simulink model "FullFMS_2026_02_17_V0_3_8"  (R2025b)
settings: Solver=ode23tb  StartTime=0.0  StopTime=inf  MaxStep=0.1  RelTol=1e-2
PreLoadFcn:
  | load("BUS_CONFIG.mat")
libraries: opcualib x8
(part 4 of 4)

== matlab function FullFMS_2026_02_17_V0_3_8/Control_20 ==
  data: u1 input; u2 input; u3 input; u4 input; u5 input; u6 input; u7 input; u8 input; u9 input; u10 input; u11 input; u12 input; C_24_CRoute_In output; C_25_CRoute_In output; C_26_CRoute_In output; C_27_CRoute_In output; C_28_CRoute_In output; C_29_CRoute_In output; C_24_Request output; C_24_CartDel output; C_24_CRoute_Out output; C_25_Request output; C_25_CartDel output; C_25_CRoute_Out output; C_26_Request output; C_26_CartDel output; C_26_CRoute_Out output; C_27_Request output; C_27_CartDel output; C_27_CRoute_Out output; C_28_Request output; C_28_CartDel output; C_28_CRoute_Out output; C_29_Request output; C_29_CartDel output; C_29_CRoute_Out output; u13 input; u14 input; u15 input; u16 input; u17 input; u18 input; u19 input; u20 input; u21 input; u22 input; u23 input; u24 input
function [C_24_CRoute_In,C_25_CRoute_In,C_26_CRoute_In,C_27_CRoute_In,...
C_28_CRoute_In,C_29_CRoute_In,C_24_Request,C_24_CartDel,C_24_CRoute_Out,...
C_25_Request,C_25_CartDel,C_25_CRoute_Out,C_26_Request,C_26_CartDel,...
C_26_CRoute_Out,C_27_Request,C_27_CartDel,C_27_CRoute_Out,C_28_Request,...
C_28_CartDel,C_28_CRoute_Out,C_29_Request,C_29_CartDel,C_29_CRoute_Out]...
= fcn_Control(u1,u2,u3,u4,u5,u6,u7,u8,u9,u10,u11,u12,u13,u14,u15,u16,...
u17,u18,u19,u20,u21,u22,u23,u24)

C_24_CRoute_In = u1;
C_25_CRoute_In = u2;
C_26_CRoute_In = u3;
C_27_CRoute_In = u4;
C_28_CRoute_In = u5;
C_29_CRoute_In = u6;
C_24_Request = u7;
C_24_CartDel = u8;
C_24_CRoute_Out = u9;
C_25_Request = u10;
C_25_CartDel = u11;
C_25_CRoute_Out = u12;
C_26_Request = u13;
C_26_CartDel = u14;
C_26_CRoute_Out = u15;
C_27_Request = u16;
C_27_CartDel = u17;
C_27_CRoute_Out = u18;
C_28_Request = u19;
C_28_CartDel = u20;
C_28_CRoute_Out = u21;
C_29_Request = u22;
C_29_CartDel = u23;
C_29_CRoute_Out = u24;

== matlab function FullFMS_2026_02_17_V0_3_8/Feedback_20 ==
  data: u1 input; F_22_Led_On output; u2 input; u3 input; u4 input; u5 input; u6 input; u7 input; u8 input; u9 input; F_22_Led_Off output; F_22_Conveyor output; F_24_Release_FB output; F_25_Release_FB output; F_26_Release_FB output; F_27_Release_FB output; F_28_Release_FB output; F_29_Release_FB output
function [F_22_Led_On,F_22_Led_Off,F_22_Conveyor,F_24_Release_FB,...
    F_25_Release_FB,F_26_Release_FB,F_27_Release_FB,F_28_Release_FB,...
    F_29_Release_FB] = fcn_Feedback(u1,u2,u3,u4,u5,u6,u7,u8,u9)

F_22_Led_On = u1;
F_22_Led_Off = u2;
F_22_Conveyor = u3;
F_24_Release_FB = u4;
F_25_Release_FB = u5;
F_26_Release_FB = u6;
F_27_Release_FB = u7;
F_28_Release_FB = u8;
F_29_Release_FB = u9;

== matlab function FullFMS_2026_02_17_V0_3_8/Sensors_20 ==
  data: u1 input; O_20_On output; u2 input; u3 input; u4 input; u5 input; u6 input; u7 input; u8 input; u9 input; u10 input; u11 input; u12 input; u13 input; u14 input; u15 input; u16 input; u17 input; u18 input; u19 input; u20 input; u21 input; u22 input; u23 input; u24 input; u25 input; u26 input; u27 input; u28 input; u29 input; u30 input; u31 input; u32 input; u33 input; O_20_Off output; O_20_Controler_On output; O_24_Cart_Stat output; O_24_Cart_Next output; O_24_Optic output; O_24_Count output; O_24_Pist_Bck output; O_25_Cart_Stat output; O_25_Cart_Next output; O_25_Optic output; O_25_Count output; O_25_Pist_Back output; O_26_Cart_Stat output; O_26_Cart_Next output; O_26_Optic output; O_26_Count output; O_26_Pist_Back output; O_27_Cart_Stat output; O_27_Cart_Next output; O_27_Optic output; O_27_Count output; O_27_Pist_Back output; O_28_Cart_Stat output; O_28_Cart_Next output; O_28_Optic output; O_28_Count output; O_28_Pist_Back output; O_29_Cart_Stat output; O_29_Cart_Next output; O_29_Optic output; O_29_Count output; O_29_Pist_Back output
function [O_20_On,O_20_Off,O_20_Controler_On,...
    O_24_Cart_Stat,O_24_Cart_Next,O_24_Optic,O_24_Count,O_24_Pist_Bck,...
    O_25_Cart_Stat,O_25_Cart_Next,O_25_Optic,O_25_Count,O_25_Pist_Back,...
    O_26_Cart_Stat,O_26_Cart_Next,O_26_Optic,O_26_Count,O_26_Pist_Back,...
    O_27_Cart_Stat,O_27_Cart_Next,O_27_Optic,O_27_Count,O_27_Pist_Back,...
    O_28_Cart_Stat,O_28_Cart_Next,O_28_Optic,O_28_Count,O_28_Pist_Back,...
    O_29_Cart_Stat,O_29_Cart_Next,O_29_Optic,O_29_Count,O_29_Pist_Back...
    ] = fcn_Sensors(u1,u2,u3,u4,u5,u6,u7,u8,u9,u10,u11,u12,u13,u14,...
    u15,u16,u17,u18,u19,u20,u21,u22,u23,u24,u25,u26,u27,u28,u29,u30,...
    u31,u32,u33)

O_20_On            = u1;
O_20_Off           = u2;
O_20_Controler_On  = u3;

O_24_Cart_Stat     = u4;
O_24_Cart_Next     = u5;
O_24_Optic         = u6;
O_24_Count         = u7;
O_24_Pist_Bck      = u8;

O_25_Cart_Stat     = u9;
O_25_Cart_Next     = u10;
O_25_Optic         = u11;
O_25_Count         = u12;
O_25_Pist_Back     = u13;

O_26_Cart_Stat     = u14;
O_26_Cart_Next     = u15;
O_26_Optic         = u16;
O_26_Count         = u17;
O_26_Pist_Back     = u18;

O_27_Cart_Stat     = u19;
O_27_Cart_Next     = u20;
O_27_Optic         = u21;
O_27_Count         = u22;
O_27_Pist_Back     = u23;

O_28_Cart_Stat     = u24;
O_28_Cart_Next     = u25;
O_28_Optic         = u26;
O_28_Count         = u27;
O_28_Pist_Back     = u28;

O_29_Cart_Stat     = u29;
O_29_Cart_Next     = u30;
O_29_Optic         = u31;
O_29_Count         = u32;
O_29_Pist_Back     = u33;

== matlab function FullFMS_2026_02_17_V0_3_8/AS-i_50 ==
  data: u1 input; u2 input; u3 input; u4 input; u5 input; u6 input; u7 input; u8 input; u9 input; u10 input; u11 input; u12 input; A_54_Request output; A_54_No_Cart output; A_54_Cart_Full output; A_54_CRoute_Out output; A_53_SortCartID output; A_54_Cart_Stat output; A_54_Cart_Next output; A_54_Optic output; A_54_Count output; A_54_Pist_Bck output; A_54_Release_FB output; A_54_CRoute_In output
function [A_54_Request, A_54_No_Cart, A_54_Cart_Full, A_54_CRoute_Out,...
A_53_SortCartID, A_54_Cart_Stat, A_54_Cart_Next, A_54_Optic, A_54_Count,...
A_54_Pist_Bck, A_54_Release_FB, A_54_CRoute_In]...
= fcn_Asi(u1,u2,u3,u4,u5,u6,u7,u8,u9,u10,u11,u12)

A_54_Request = u1;
A_54_No_Cart = u2;
A_54_Cart_Full = u3;
A_54_CRoute_Out = u4;
A_53_SortCartID = u5;
A_54_Cart_Stat = u6;
A_54_Cart_Next = u7;
A_54_Optic = u8;
A_54_Count = u9;
A_54_Pist_Bck = u10;
A_54_Release_FB = u11;
A_54_CRoute_In = u12;

== matlab function FullFMS_2026_02_17_V0_3_8/Control_50 ==
  data: u1 input; C_55_Initialization output; u2 input; u3 input; u4 input; u5 input; C_55_PD_Sort output; C_52_Profibus output; C_55_Start output; C_55_Cart2Del output
function [C_55_Initialization,C_55_PD_Sort,C_52_Profibus,...
    C_55_Start,C_55_Cart2Del] = fcn_Control(u1,u2,u3,u4,u5)

C_55_Initialization = u1;
C_55_PD_Sort = u2;
C_52_Profibus = u3;
C_55_Start = u4;
C_55_Cart2Del = u5;

== matlab function FullFMS_2026_02_17_V0_3_8/Feedback_50 ==
  data: u1 input; F_52_Claw_2_Del output; u2 input; u3 input; u4 input; u5 input; u6 input; u7 input; u8 input; u9 input; u10 input; u11 input; u12 input; F_52_Claw_2_Cart output; F_52_Claw_Down output; F_52_Close_Claw output; F_53_Led_Start output; F_53_Led_Reset output; F_53_Led_Extra1 output; F_53_Led_Extra2 output; F_53_Panel_O4 output; F_53_Panel_O5 output; F_53_Panel_O6 output; F_53_Panel_O7 output
function [F_52_Claw_2_Del,F_52_Claw_2_Cart,F_52_Claw_Down,...
    F_52_Close_Claw,F_53_Led_Start,F_53_Led_Reset,F_53_Led_Extra1,...
    F_53_Led_Extra2,F_53_Panel_O4,F_53_Panel_O5,F_53_Panel_O6,...
    F_53_Panel_O7] = fcn_Feedback(u1,u2,u3,u4,u5,u6,u7,u8,u9,u10,u11,u12)

F_52_Claw_2_Del = u1;
F_52_Claw_2_Cart = u2;
F_52_Claw_Down = u3;
F_52_Close_Claw = u4;
F_53_Led_Start = u5;
F_53_Led_Reset = u6;
F_53_Led_Extra1 = u7;
F_53_Led_Extra2 = u8;
F_53_Panel_O4 = u9;
F_53_Panel_O5 = u10;
F_53_Panel_O6 = u11;
F_53_Panel_O7 = u12;

== matlab function FullFMS_2026_02_17_V0_3_8/Sensors_50 ==
  data: u1 input; O_50_Part_Reserve output; u2 input; u3 input; u4 input; u5 input; u6 input; u7 input; u8 input; u9 input; u10 input; u11 input; u12 input; u13 input; u14 input; u15 input; O_50_Claw_Cart output; O_50_Claw_Del output; O_50_Claw_Reserve output; O_50_Claw_Low output; O_50_Claw_High output; O_50_Part_in_Claw output; O_51_Start output; O_51_Stop output; O_51_Key_Pos output; O_51_Reset output; O_51_Panel_I4 output; O_51_Panel_I5 output; O_51_Panel_I6 output; O_51_Panel_I7 output
function [O_50_Part_Reserve,O_50_Claw_Cart,O_50_Claw_Del,...
    O_50_Claw_Reserve,O_50_Claw_Low,O_50_Claw_High,O_50_Part_in_Claw,...
    O_51_Start,O_51_Stop,O_51_Key_Pos,O_51_Reset,O_51_Panel_I4,...
    O_51_Panel_I5,O_51_Panel_I6,O_51_Panel_I7] = fcn_Sensors(u1,u2,u3,u4,...
    u5,u6,u7,u8,u9,u10,u11,u12,u13,u14,u15)

O_50_Part_Reserve = u1;
O_50_Claw_Cart = u2;
O_50_Claw_Del = u3;
O_50_Claw_Reserve = u4;
O_50_Claw_Low = u5;
O_50_Claw_High = u6;
O_50_Part_in_Claw = u7;
O_51_Start = u8;
O_51_Stop = u9;
O_51_Key_Pos = u10;
O_51_Reset = u11;
O_51_Panel_I4 = u12;
O_51_Panel_I5 = u13;
O_51_Panel_I6 = u14;
O_51_Panel_I7 = u15;

== matlab function FullFMS_2026_02_17_V0_3_8/AS-i_90 ==
  data: u1 input; A_94_Request output; u2 input; u3 input; u4 input; u5 input; u6 input; u7 input; u8 input; u9 input; A_94_No_Cart output; A_94_Cart_Full output; A_94_CRoute_Out output; A_93_ProcCartID output; A_94_Cart_Stat output; A_94_Cart_Next output; A_94_Optic output; A_94_Count output; A_94_Pist_Bck output; A_94_Release_FB output; u10 input; u11 input; u12 input; A_94_CRoute_In output
function [A_94_Request,A_94_No_Cart,A_94_Cart_Full,A_94_CRoute_Out,...
A_93_ProcCartID,A_94_Cart_Stat,A_94_Cart_Next,A_94_Optic,A_94_Count,...
A_94_Pist_Bck,A_94_Release_FB,A_94_CRoute_In]...
= fcn_Asi(u1,u2,u3,u4,u5,u6,u7,u8,u9,u10,u11,u12)

A_94_Request = u1;
A_94_No_Cart = u2;
A_94_Cart_Full = u3;
A_94_CRoute_Out = u4;
A_93_ProcCartID = u5;
A_94_Cart_Stat = u6;
A_94_Cart_Next = u7;
A_94_Optic = u8;
A_94_Count = u9;
A_94_Pist_Bck = u10;
A_94_Release_FB = u11;
A_94_CRoute_In = u12;

== matlab function FullFMS_2026_02_17_V0_3_8/Control_90 ==
  data: C_95_Initialization output; C_95_PD_Proc output; C_95_PD_Cart output; u1 input; C_92_Profibus output; u2 input; u3 input; u4 input; u5 input; C_95_Start output; C_95_Cart2Del output; C_95_Del2Cart output; u6 input; u7 input
function [C_95_Initialization,C_95_PD_Proc,C_95_PD_Cart,C_92_Profibus,...
C_95_Start,C_95_Cart2Del,C_95_Del2Cart]...
= fcn_Control(u1,u2,u3,u4,u5,u6,u7)

C_95_Initialization = u1;
C_95_PD_Proc = u2;
C_95_PD_Cart = u3;
C_92_Profibus = u4;
C_95_Start = u5;
C_95_Cart2Del = u6;
C_95_Del2Cart = u7;

== matlab function FullFMS_2026_02_17_V0_3_8/Feedback_90 ==
  data: u1 input; F_92_Claw_2_Cart output; u2 input; u3 input; u4 input; u5 input; u6 input; u7 input; u8 input; u9 input; u10 input; u11 input; u12 input; F_92_Claw_2_Del output; F_92_Claw_Down output; F_92_Close_Claw output; F_93_Led_Start output; F_93_Led_Reset output; F_93_Led_Extra1 output; F_93_Led_Extra2 output; F_93_Panel_O4 output; F_93_Panel_O5 output; F_93_Panel_O6 output; F_93_Panel_O7 output
function [F_92_Claw_2_Cart,F_92_Claw_2_Del,F_92_Claw_Down,...
    F_92_Close_Claw,F_93_Led_Start,F_93_Led_Reset,F_93_Led_Extra1,...
    F_93_Led_Extra2,F_93_Panel_O4,F_93_Panel_O5,F_93_Panel_O6,...
    F_93_Panel_O7] = fcn_Feedback(u1,u2,u3,u4,u5,u6,u7,u8,u9,u10,u11,u12)

F_92_Claw_2_Cart = u1;
F_92_Claw_2_Del = u2;
F_92_Claw_Down = u3;
F_92_Close_Claw = u4;
F_93_Led_Start = u5;
F_93_Led_Reset = u6;
F_93_Led_Extra1 = u7;
F_93_Led_Extra2 = u8;
F_93_Panel_O4 = u9;
F_93_Panel_O5 = u10;
F_93_Panel_O6 = u11;
F_93_Panel_O7 = u12;

== matlab function FullFMS_2026_02_17_V0_3_8/Sensors_90 ==
  data: u1 input; O_90_Part_Reserve output; u2 input; u3 input; u4 input; u5 input; u6 input; u7 input; u8 input; u9 input; u10 input; u11 input; u12 input; u13 input; u14 input; u15 input; O_90_Claw_Del output; O_90_Claw_Cart output; O_90_Claw_Reserve output; O_90_Claw_Low output; O_90_Claw_High output; O_90_Part_in_Claw output; O_91_Start output; O_91_Stop output; O_91_Key_Pos output; O_91_Reset output; O_91_Panel_I4 output; O_91_Panel_I5 output; O_91_Panel_I6 output; O_91_Panel_I7 output
function [O_90_Part_Reserve,O_90_Claw_Del,O_90_Claw_Cart,...
    O_90_Claw_Reserve,O_90_Claw_Low,O_90_Claw_High,O_90_Part_in_Claw,...
    O_91_Start,O_91_Stop,O_91_Key_Pos,O_91_Reset,O_91_Panel_I4,...
    O_91_Panel_I5,O_91_Panel_I6,O_91_Panel_I7] = fcn_Sensors(u1,u2,u3,u4,...
    u5,u6,u7,u8,u9,u10,u11,u12,u13,u14,u15)

O_90_Part_Reserve = u1;
O_90_Claw_Del = u2;
O_90_Claw_Cart = u3;
O_90_Claw_Reserve = u4;
O_90_Claw_Low = u5;
O_90_Claw_High = u6;
O_90_Part_in_Claw = u7;
O_91_Start = u8;
O_91_Stop = u9;
O_91_Key_Pos = u10;
O_91_Reset = u11;
O_91_Panel_I4 = u12;
O_91_Panel_I5 = u13;
O_91_Panel_I6 = u14;
O_91_Panel_I7 = u15;

== matlab function FullFMS_2026_02_17_V0_3_8/Control_100 ==
  data: C_105_Initialization output; C_105_Part_ready output; C_105_Test_Ok output; C_105_Test_Fail output; u1 input; C_102_Profibus output boolean; C_103_RQ_Turns output; u2 input; u3 input; u4 input; u5 input; u6 input; u7 input; C_105_Start output; C_105_Test output; C_105_TestDrill output; C_105_Rotation output; u8 input; u9 input; u10 input
function [C_105_Initialization, C_105_Part_ready, C_105_Test_Ok,...
C_105_Test_Fail, C_102_Profibus, C_103_RQ_Turns, C_105_Start,...
C_105_Test, C_105_TestDrill, C_105_Rotation] = fcn_Control(u1,u2,u3,u4,...
u5,u6,u7,u8,u9,u10)

C_105_Initialization = u1;
C_105_Part_ready = u2;
C_105_Test_Ok = u3;
C_105_Test_Fail = u4;
C_102_Profibus = u5;
C_103_RQ_Turns = u6;
C_105_Start = u7;
C_105_Test = u8;
C_105_TestDrill = u9;
C_105_Rotation = u10;

== matlab function FullFMS_2026_02_17_V0_3_8/Feedback_100 ==
  data: u1 input; F_102_Drill_On output; u2 input; u3 input; u4 input; u5 input; u6 input; u7 input; u8 input; u9 input; u10 input; u11 input; u12 input; u13 input; u14 input; F_102_RT_On output; F_102_Drill_Down output; F_102_Drill_Up output; F_102_Drill_Pin output; F_102_Test_Pin output; F_103_Led_Start output; F_103_Led_Reset output; F_103_Led_Extra1 output; F_103_Led_Extra2 output; F_103_Panel_O4 output; F_103_Panel_O5 output; F_103_Panel_O6 output; F_103_Panel_O7 output
function [F_102_Drill_On, F_102_RT_On, F_102_Drill_Down, F_102_Drill_Up,...
          F_102_Drill_Pin, F_102_Test_Pin,F_103_Led_Start,...
          F_103_Led_Reset, F_103_Led_Extra1, F_103_Led_Extra2,...
          F_103_Panel_O4, F_103_Panel_O5, F_103_Panel_O6, F_103_Panel_O7] = ...
          fcn_Feedback(u1,u2,u3,u4,u5,u6,u7,u8,u9,u10,u11,u12,u13,u14)

F_102_Drill_On   = u1;
F_102_RT_On      = u2;
F_102_Drill_Down = u3;
F_102_Drill_Up   = u4;
F_102_Drill_Pin  = u5;
F_102_Test_Pin   = u6;

F_103_Led_Start  = u7;
F_103_Led_Reset  = u8;
F_103_Led_Extra1 = u9;
F_103_Led_Extra2 = u10;

F_103_Panel_O4   = u11;
F_103_Panel_O5   = u12;
F_103_Panel_O6   = u13;
F_103_Panel_O7   = u14;

== matlab function FullFMS_2026_02_17_V0_3_8/Sensors_100 ==
  data: u1 input; O_100_PInit_Pos output; u2 input; u3 input; u4 input; u5 input; u6 input; u7 input; u8 input; u9 input; u10 input; u11 input; u12 input; u13 input; u14 input; u15 input; O_100_PDrill_Pos output; O_100_PTest_Pos output; O_100_SDrill_High output; O_100_SDrill_Low output; O_100_RT_Sensor output; O_100_PTest_Ok output; O_101_Start output; O_101_Stop output; O_101_Key_Pos output; O_101_Reset output; O_101_Panel_I4 output; O_101_Panel_I5 output; O_101_Panel_I6 output; O_101_Panel_I7 output
function [O_100_PInit_Pos, O_100_PDrill_Pos, O_100_PTest_Pos, ...
          O_100_SDrill_High, O_100_SDrill_Low, O_100_RT_Sensor,...
          O_100_PTest_Ok,O_101_Start, O_101_Stop, O_101_Key_Pos,...
          O_101_Reset,O_101_Panel_I4, O_101_Panel_I5, O_101_Panel_I6,...
          O_101_Panel_I7] = fcn_Sensors(u1,u2,u3,u4,u5,u6,u7,u8,u9,u10,...
          u11,u12,u13,u14,u15)

    O_100_PInit_Pos   = u1;
    O_100_PDrill_Pos  = u2;
    O_100_PTest_Pos   = u3;
    O_100_SDrill_High = u4;
    O_100_SDrill_Low  = u5;
    O_100_RT_Sensor   = u6;
    O_100_PTest_Ok    = u7;

    O_101_Start       = u8;
    O_101_Stop        = u9;
    O_101_Key_Pos     = u10;
    O_101_Reset       = u11;

    O_101_Panel_I4    = u12;
    O_101_Panel_I5    = u13;
    O_101_Panel_I6    = u14;
    O_101_Panel_I7    = u15;

== matlab function FullFMS_2026_02_17_V0_3_8/AS-i_30 ==
  data: u1 input; A_34_Request output; u2 input; u3 input; u4 input; u5 input; u6 input; u7 input; u8 input; u9 input; A_34_No_Cart output; A_34_Cart_Full output; A_34_CRoute_Out output; A_32_RoboCartID output; A_34_Cart_Stat output; A_34_Cart_Next output; A_34_Optic output; A_34_Count output; A_34_Pist_Bck output; A_34_Release_FB output; u10 input; u11 input; u12 input; A_34_CRoute_In output
function [A_34_Request,A_34_No_Cart,A_34_Cart_Full,A_34_CRoute_Out,...
A_32_RoboCartID,A_34_Cart_Stat,A_34_Cart_Next,A_34_Optic,A_34_Count,...
A_34_Pist_Bck,A_34_Release_FB,A_34_CRoute_In]... 
= fcn_Asi(u1,u2,u3,u4,u5,u6,u7,u8,u9,u10,u11,u12)

A_34_Request = u1;
A_34_No_Cart = u2;
A_34_Cart_Full = u3;
A_34_CRoute_Out = u4;
A_32_RoboCartID = u5;
A_34_Cart_Stat = u6;
A_34_Cart_Next = u7;
A_34_Optic = u8;
A_34_Count = u9;
A_34_Pist_Bck = u10;
A_34_Release_FB = u11;
A_34_CRoute_In = u12;

== matlab function FullFMS_2026_02_17_V0_3_8/Control_30 ==
  data: C_35_Part_Del output; C_30_Robot1 output; C_30_Robot2 output; u1 input; u2 input; u3 input
function [C_35_Part_Del,C_30_Robot1,C_30_Robot2] = fcn_Control(u1,u2,u3)

C_35_Part_Del = u1;
C_30_Robot1 = u2;
C_30_Robot2 = u3;

== matlab function FullFMS_2026_02_17_V0_3_8/Feedback_30 ==
  data: u1 input; F_33_Led_Start output; u2 input; u3 input; u4 input; u5 input; u6 input; F_33_Led_Reset output; F_33_Led_Extra1 output; F_33_Led_Extra2 output; F_33_Spring_Cyl output; F_33_Cover_Cyl output
function [F_33_Led_Start,F_33_Led_Reset,...
    F_33_Led_Extra1,F_33_Led_Extra2,...
    F_33_Spring_Cyl,F_33_Cover_Cyl] = fcn_Feedback(u1,u2,u3,u4,u5,u6)

F_33_Led_Start = u1
F_33_Led_Reset = u2
F_33_Led_Extra1 = u3
F_33_Led_Extra2 = u4
F_33_Spring_Cyl = u5
F_33_Cover_Cyl = u6

== matlab function FullFMS_2026_02_17_V0_3_8/Control_60 ==
  data: u1 input; C_65_Initialization output; u2 input; u3 input; u4 input; u5 input; u6 input; u7 input; u8 input; u9 input; u10 input; C_65_ID_1 output; C_65_ID_2 output; C_65_Part_Sorted output; C_62_Profibus output; C_65_RBS_Output output; C_65_RSB_Output output; C_65_BRS_Output output; C_65_BSR_Output output; C_65_SRB_Output output; C_65_SBR_Output output; u11 input
function [C_65_Initialization, C_65_ID_1, C_65_ID_2, C_65_Part_Sorted, ...
          C_62_Profibus,C_65_RBS_Output, C_65_RSB_Output, ...
          C_65_BRS_Output, C_65_BSR_Output,C_65_SRB_Output,... 
          C_65_SBR_Output] = ...
          fcn_Control(u1,u2,u3,u4,u5,u6,u7,u8,u9,u10,u11)

    C_65_Initialization = u1;
    C_65_ID_1           = u2;
    C_65_ID_2           = u3;
    C_65_Part_Sorted    = u4;
    C_62_Profibus       = u5;
    C_65_RBS_Output     = u6;
    C_65_RSB_Output     = u7;
    C_65_BRS_Output     = u8;
    C_65_BSR_Output     = u9;
    C_65_SRB_Output     = u10;
    C_65_SBR_Output     = u11;

== matlab function FullFMS_2026_02_17_V0_3_8/Sensors_30 ==
  data: u1 input; O_31_Start output; u2 input; u3 input; u4 input; u5 input; u6 input; u7 input; u8 input; u9 input; u10 input; u11 input; u12 input; O_31_Stop output; O_31_Reset output; O_31_Part_in_Claw output; O_31_Orientation output; O_32_Sp_Cyl_Bck output; O_32_Sp_Cyl_Fwd output; O_32_Co_Cyl_Bck output; O_32_Co_Cyl_Fwd output; O_32_Sp_PickUp output; O_32_Co_PickUp output; O_32_CoMag_Empty output
function [O_31_Start,...
    O_31_Stop,O_31_Reset,...
    O_31_Part_in_Claw,O_31_Orientation,...
    O_32_Sp_Cyl_Bck,O_32_Sp_Cyl_Fwd,...
    O_32_Co_Cyl_Bck,O_32_Co_Cyl_Fwd,...
    O_32_Sp_PickUp,O_32_Co_PickUp,...
    O_32_CoMag_Empty] = fcn_Sensors(u1,u2,u3,u4,u5,u6,u7,u8,u9,u10,u11,u12)

O_31_Start = u1
O_31_Stop = u2
O_31_Reset = u3
O_31_Part_in_Claw = u4
O_31_Orientation = u5
O_32_Sp_Cyl_Bck = u6
O_32_Sp_Cyl_Fwd = u7
O_32_Co_Cyl_Bck = u8
O_32_Co_Cyl_Fwd = u9
O_32_Sp_PickUp = u10
O_32_Co_PickUp = u11
O_32_CoMag_Empty = u12

== matlab function FullFMS_2026_02_17_V0_3_8/Feedback_60 ==
  data: u1 input; F_62_Conveyor output; u2 input; u3 input; u4 input; u5 input; u6 input; u7 input; u8 input; u9 input; u10 input; u11 input; u12 input; F_62_P1 output; F_62_P2 output; F_62_Identify output; F_63_Led_Start output; F_63_Led_Reset output; F_63_Led_Extra1 output; F_63_Led_Extra2 output; F_63_Panel_O4 output; F_63_Panel_O5 output; F_63_Panel_O6 output; F_63_Panel_O7 output
function [F_62_Conveyor, F_62_P1, F_62_P2, F_62_Identify, ...
          F_63_Led_Start, F_63_Led_Reset, F_63_Led_Extra1, F_63_Led_Extra2, ...
          F_63_Panel_O4, F_63_Panel_O5, F_63_Panel_O6, F_63_Panel_O7] = ...
          fcn_Feedback(u1,u2,u3,u4,u5,u6,u7,u8,u9,u10,u11,u12)

    F_62_Conveyor   = u1;
    F_62_P1         = u2;
    F_62_P2         = u3;
    F_62_Identify   = u4;

    F_63_Led_Start  = u5;
    F_63_Led_Reset  = u6;
    F_63_Led_Extra1 = u7;
    F_63_Led_Extra2 = u8;

    F_63_Panel_O4   = u9;
    F_63_Panel_O5   = u10;
    F_63_Panel_O6   = u11;
    F_63_Panel_O7   = u12;

== matlab function FullFMS_2026_02_17_V0_3_8/Sensors_60 ==
  data: u1 input; O_60_SPart output; u2 input; u3 input; u4 input; u5 input; u6 input; u7 input; u8 input; u9 input; u10 input; u11 input; u12 input; u13 input; u14 input; u15 input; u16 input; O_60_Slnd output; O_60_SPhoto output; O_60_Part_Pass output; O_60_SL1_Bck output; O_60_SL1_Fwd output; O_60_SL2_Bck output; O_60_SL2_Fwd output; O_61_Start output; O_61_Stop output; O_61_Key_Pos output; O_61_Reset output; O_61_Panel_I4 output; O_61_Panel_I5 output; O_61_Panel_I6 output; O_61_Panel_I7 output
function [ ...
    O_60_SPart, O_60_Slnd, O_60_SPhoto, O_60_Part_Pass, ...
    O_60_SL1_Bck, O_60_SL1_Fwd, O_60_SL2_Bck, O_60_SL2_Fwd, ...
    O_61_Start, O_61_Stop, O_61_Key_Pos, O_61_Reset, ...
    O_61_Panel_I4, O_61_Panel_I5, O_61_Panel_I6, O_61_Panel_I7] = ...
    fcn_Sensors(u1,u2,u3,u4,u5,u6,u7,u8,u9,u10,u11,u12,u13,u14,u15,u16)

O_60_SPart      = u1;
O_60_Slnd       = u2;
O_60_SPhoto     = u3;
O_60_Part_Pass  = u4;

O_60_SL1_Bck    = u5;
O_60_SL1_Fwd    = u6;
O_60_SL2_Bck    = u7;
O_60_SL2_Fwd    = u8;

O_61_Start      = u9;
O_61_Stop       = u10;
O_61_Key_Pos    = u11;
O_61_Reset      = u12;

O_61_Panel_I4   = u13;
O_61_Panel_I5   = u14;
O_61_Panel_I6   = u15;
O_61_Panel_I7   = u16;

== matlab function FullFMS_2026_02_17_V0_3_8/AS-i_40 ==
  data: u1 input; u2 input; u3 input; u4 input; u5 input; u6 input; u7 input; u8 input; u9 input; u10 input; u11 input; A_44_Request output; A_44_No_Cart output; A_44_Cart_Full output; A_44_CRoute_In output; A_43_StorCartID output; A_44_Cart_Stat output; A_44_Cart_Next output; A_44_Optic output; A_44_Count output; A_44_Pist_Bck output; A_44_Release_FB output; A_44_CRoute_Out output; u12 input
function [A_44_Request,A_44_No_Cart, A_44_Cart_Full, A_44_CRoute_In,...
A_43_StorCartID, A_44_Cart_Stat, A_44_Cart_Next, A_44_Optic, A_44_Count,...
A_44_Pist_Bck,A_44_Release_FB, A_44_CRoute_Out] = ...
fcn_Asi_store(u1,u2,u3,u4,u5,u6,u7,u8,u9,u10,u11,u12)

A_44_Request = u1;
A_44_No_Cart = u2;
A_44_Cart_Full = u3;
A_44_CRoute_In = u4;
A_43_StorCartID = u5;
A_44_Cart_Stat = u6;
A_44_Cart_Next = u7;
A_44_Optic = u8;
A_44_Count = u9;
A_44_Pist_Bck = u10;
A_44_Release_FB = u11;
A_44_CRoute_Out = u12;

== matlab function FullFMS_2026_02_17_V0_3_8/Control_40 ==
  data: u1 input; u2 input; u3 input; u4 input; u5 input; C_45_Initialization output; C_42_Profibus output; C_45_Start output; C_45_StorePart output; C_45_RetrievePart output
function [C_45_Initialization, C_42_Profibus, C_45_Start, C_45_StorePart,...
C_45_RetrievePart] = fcn_Control_Storage(u1,u2,u3,u4,u5)

C_45_Initialization = u1;
C_42_Profibus = u2;
C_45_Start = u3;
C_45_StorePart = u4;
C_45_RetrievePart = u5;

== matlab function FullFMS_2026_02_17_V0_3_8/Feedback_40 ==
  data: u1 input; F_43_Led_Start output; u2 input; u3 input; u4 input; u5 input; u6 input; u7 input; u8 input; F_43_Led_Reset output; F_43_Led_Extra1 output; F_43_Led_Extra2 output; F_43_Panel_O4 output; F_43_Panel_O5 output; F_43_Panel_O6 output; F_43_Panel_O7 output
function [F_43_Led_Start, F_43_Led_Reset, F_43_Led_Extra1, F_43_Led_Extra2,...
F_43_Panel_O4, F_43_Panel_O5, F_43_Panel_O6, F_43_Panel_O7] = ...
fcn_feedback_storage(u1,u2,u3,u4,u5,u6,u7,u8)

F_43_Led_Start = u1;
F_43_Led_Reset = u2;
F_43_Led_Extra1 = u3;
F_43_Led_Extra2 = u4;
F_43_Panel_O4 = u5;
F_43_Panel_O5 = u6;
F_43_Panel_O6 = u7;
F_43_Panel_O7 = u8;

== matlab function FullFMS_2026_02_17_V0_3_8/Sensors_40 ==
  data: u1 input; O_41_Start output; u2 input; u3 input; u4 input; u5 input; u6 input; u7 input; u8 input; O_41_Stop output; O_41_Key_Pos output; O_41_Reset output; O_41_Panel_I4 output; O_41_Panel_I5 output; O_41_Panel_I6 output; O_41_Panel_I7 output
function [O_41_Start, O_41_Stop, O_41_Key_Pos, O_41_Reset, O_41_Panel_I4,...
O_41_Panel_I5, O_41_Panel_I6, O_41_Panel_I7] = fcn_sensors_40(u1,u2,u3,u4,u5,u6,u7,u8)

O_41_Start = u1;
O_41_Stop = u2;
O_41_Key_Pos = u3;
O_41_Reset = u4;
O_41_Panel_I4 = u5;
O_41_Panel_I5 = u6;
O_41_Panel_I6 = u7;
O_41_Panel_I7 = u8;
